simulink model "dsm_mash_2_1_ciff_10mhz_topology_model"  (R2025b)
settings: Solver=FixedStepDiscrete  StartTime=0.0  StopTime=0.0008191  FixedStep=1e-07  RelTol=1e-3
model workspace (MAT data in the model file):
  A1_mash = [1  0; 1  1]
  A2_mash = 1
  B1_mash = [1  -1; 0  0]
  B2_mash = [1 -1]
  C1_mash = [1.23606797746 0.472135954976]
  C2_mash = 0.666666666641
  D1_mash = [1 0]
  D2_mash = [1 0]
  Ts_mash = 1e-07
  n_stages_mash = 2
undefined symbols (not defined in the file or in its folder): dsm_quantizer
settings Model: Creator=sli767  LastModifiedBy=sli767

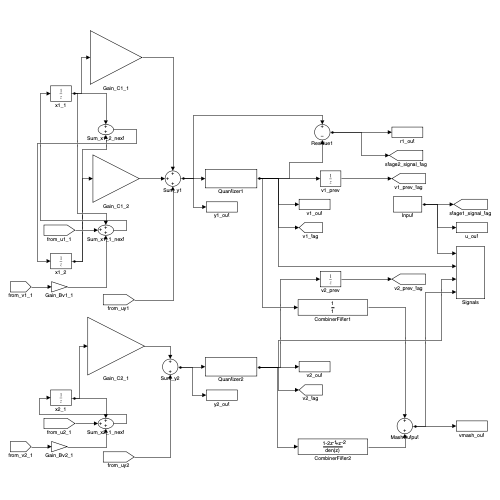
[thumbnail: Simulink's stored preview of the top-level diagram]
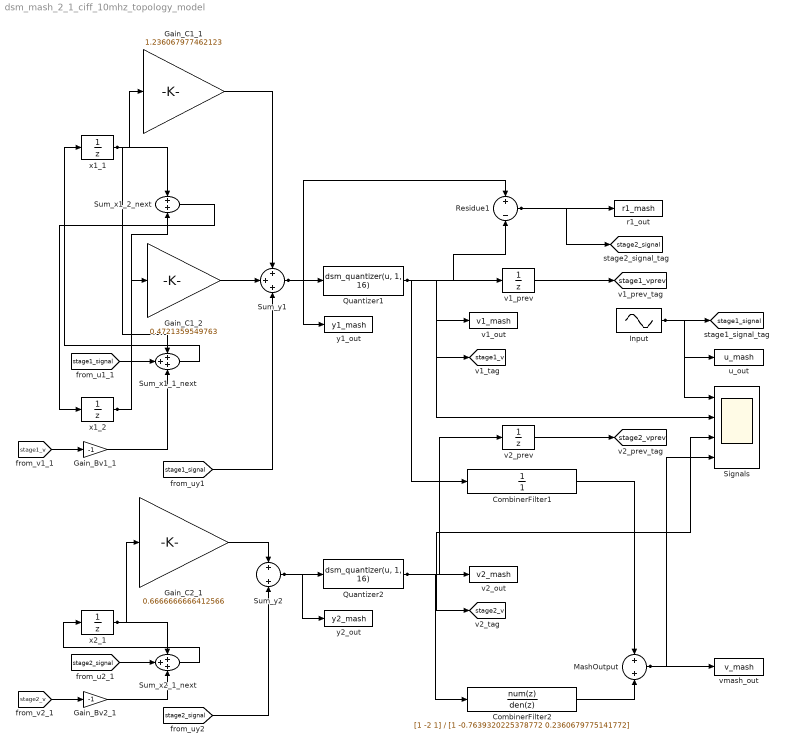
== system dsm_mash_2_1_ciff_10mhz_topology_model ==
  CombinerFilter1 : DiscreteFilter  Numerator=1  Denominator=1
  CombinerFilter2 : DiscreteFilter  Numerator=[1 -2 1]  Denominator=[1 -0.7639320225378772 0.2360679775141772]
  Gain_Bv1_1 : Gain  Gain=-1
  Gain_Bv2_1 : Gain  Gain=-1
  Gain_C1_1 : Gain  Gain=1.236067977462123
  Gain_C1_2 : Gain  Gain=0.4721359549763
  Gain_C2_1 : Gain  Gain=0.6666666666412566
  Input : Sin  Amplitude=0.5  Frequency=368155.3890925539  SampleTime=1e-07
  MashOutput : Sum
  Quantizer1 : MATLABFcn  MATLABFcn=dsm_quantizer(u, 1, 16)
  Quantizer2 : MATLABFcn  MATLABFcn=dsm_quantizer(u, 1, 16)
  Residue1 : Sum  Inputs=+-
  Signals : Scope  NumInputPorts=4
  Sum_x1_1_next : Sum  Inputs=+++
  Sum_x1_2_next : Sum
  Sum_x2_1_next : Sum  Inputs=+++
  Sum_y1 : Sum  Inputs=+++
  Sum_y2 : Sum
  r1_out : ToWorkspace  VariableName=r1_mash  SampleTime=-1
  u_out : ToWorkspace  VariableName=u_mash  SampleTime=-1
  v1_out : ToWorkspace  VariableName=v1_mash  SampleTime=-1
  v1_prev : UnitDelay  SampleTime=Ts_mash  HasFrameUpgradeWarning=on
  v2_out : ToWorkspace  VariableName=v2_mash  SampleTime=-1
  v2_prev : UnitDelay  SampleTime=Ts_mash  HasFrameUpgradeWarning=on
  vmash_out : ToWorkspace  VariableName=v_mash  SampleTime=-1
  x1_1 : UnitDelay  SampleTime=Ts_mash  HasFrameUpgradeWarning=on
  x1_2 : UnitDelay  SampleTime=Ts_mash  HasFrameUpgradeWarning=on
  x2_1 : UnitDelay  SampleTime=Ts_mash  HasFrameUpgradeWarning=on
  y1_out : ToWorkspace  VariableName=y1_mash  SampleTime=-1
  y2_out : ToWorkspace  VariableName=y2_mash  SampleTime=-1
  tag scope: stage1_signal=global, stage1_v=global, stage1_vprev=global, stage2_signal=global, stage2_v=global, stage2_vprev=global
  wires:
  CombinerFilter2/1 -> MashOutput/2
  v2_prev/1 -> [stage2_vprev]
  Gain_Bv2_1/1 -> Sum_x2_1_next/3
  v1_prev/1 -> [stage1_vprev]
  Input/1 -> Signals/1, [stage1_signal], u_out/1
  CombinerFilter1/1 -> MashOutput/1
  Quantizer2/1 -> CombinerFilter2/1, v2_out/1, [stage2_v], v2_prev/1, Signals/3
  Gain_C1_1/1 -> Sum_y1/1
  Sum_y2/1 -> y2_out/1, Quantizer2/1
  Sum_y1/1 -> y1_out/1, Residue1/1, Quantizer1/1
  Sum_x1_1_next/1 -> x1_1/1
  MashOutput/1 -> Signals/4, vmash_out/1
  Sum_x2_1_next/1 -> x2_1/1
  Gain_C2_1/1 -> Sum_y2/1
  Gain_C1_2/1 -> Sum_y1/2
  Sum_x1_2_next/1 -> x1_2/1
  [stage1_signal] -> Sum_x1_1_next/2
  [stage2_signal] -> Sum_x2_1_next/2
  x2_1/1 -> Gain_C2_1/1, Sum_x2_1_next/1
  [stage1_v] -> Gain_Bv1_1/1
  x1_1/1 -> Gain_C1_1/1, Sum_x1_2_next/1, Sum_x1_1_next/1
  Gain_Bv1_1/1 -> Sum_x1_1_next/3
  x1_2/1 -> Gain_C1_2/1, Sum_x1_2_next/2
  Residue1/1 -> [stage2_signal], r1_out/1
  Quantizer1/1 -> v1_out/1, Signals/2, [stage1_v], CombinerFilter1/1, v1_prev/1, Residue1/2
  [stage2_signal] -> Sum_y2/2
  [stage1_signal] -> Sum_y1/3
  [stage2_v] -> Gain_Bv2_1/1
